simulink model "heading_controller"  (R2017b)
settings: Solver=ode45  StartTime=tstart  StopTime=tstop  RelTol=1e-3  EnableMultiTasking=on
values from neighbouring files (symbols this model uses):
  c = 0    [TTK4190_A3_task1_2.m]    (also in TTK4190_A3_task1_3.m = 1; model_analysis.m; msfartoystyring.m = sqrt(cun*ur*n + cnn*n^2); sysID.m)
  delta_max = 25*deg2rad    (= 0.436332312999)    [TTK4190_A3_task1_3.m]    (also in msfartoystyring.m)
  delta_min = -25*deg2rad    (= -0.436332312999)    [TTK4190_A3_task1_3.m]
  Kd_psi = 650    [TTK4190_A3_task1_3.m]    (also in parameters_heading_controller.m = 150)
  Ki_psi = 0.07    [TTK4190_A3_task1_3.m]    (also in parameters_heading_controller.m = 0.0004)
  Kp_psi = 60    [TTK4190_A3_task1_3.m]    (also in parameters_heading_controller.m = 0.8)
  nc = 7.3    [TTK4190_A3_task1_2.m]    (also in TTK4190_A3_task1_3.m; model_analysis.m; parameters_heading_controller.m; sysID.m)
  p0 = zeros(2,1)    [TTK4190_A3_task1_2.m]    (also in TTK4190_A3_task1_3.m; model_analysis.m; sysID.m)
  psi0 = 0    [TTK4190_A3_task1_2.m]    (also in TTK4190_A3_task1_3.m; model_analysis.m; sysID.m)
  psi_amp = -0.3    [TTK4190_A3_task1_3.m]
  psi_d = 5*deg2rad    (= 0.0872664625997)    [TTK4190_A3_task1_2.m]    (also in TTK4190_A3_task1_3.m = 0.13962634016; model_analysis.m = 0.13962634016; parameters_heading_controller.m = 0.13962634016)
  psi_freq = 0.008    [TTK4190_A3_task1_3.m]
  r0 = 0    [TTK4190_A3_task1_2.m]    (also in TTK4190_A3_task1_3.m; model_analysis.m; sysID.m)
  tsamp = 10    [TTK4190_A3_task1_2.m]    (also in TTK4190_A3_task1_3.m; model_analysis.m = 35; sim_nomoto2.m = tsamp; sysID.m = 100)
  v0 = [6.63 0]'    [TTK4190_A3_task1_2.m]    (also in TTK4190_A3_task1_3.m; model_analysis.m; sysID.m)
undefined symbols (not defined in the file or in its folder): msfartoystyring
settings Model: ExtModeAutoUpdateStatusClock=off  Creator=christh  LastModifiedBy=Marie
settings DataIOCC: LimitDataPoints=on  SaveFormat=Array  SignalLoggingSaveFormat=ModelDataLogs
settings OptimizationCC: ExpressionDepthLimit=2147483647  InitFltsAndDblsToZero=on  LifeSpan=inf
settings DebuggingCC: UnderspecifiedInitializationDetection=Classic  MergeDetectMultiDrivingBlocksExec=none  SolverPrmCheckMsg=warning  FcnCallInpInsideContextMsg=warning  StateNameClashWarn=warning  SFUnexpectedBacktrackingDiag=warning  SFNoUnconditionalDefaultTransitionDiag=warning  SFExecutionAtInitializationDiag=none
settings HardwareCC: ProdBitPerPointer=32  ProdBitPerSizeT=32  ProdBitPerPtrDiffT=32  ProdLargestAtomicFloat=None  ProdIntDivRoundTo=Undefined  ProdEndianess=Unspecified  ProdWordSize=32  ProdHWDeviceType=32-bit Generic
settings ModelReferenceCC: PropagateSignalLabelsOutOfModel=off
settings CodeAppCC: StateflowObjectComments=on
settings GRTTargetCC: TargetLangStandard=C89/C90 (ANSI)  GeneratePreprocessorConditionals=Disable all  CombineOutputUpdateFcns=off  GRTInterface=on
settings ConfigComp: CovMetricSettings=dw  CovHtmlReporting=on  CovSaveCumulativeToWorkspaceVar=on  CovSaveSingleToWorkspaceVar=on  CovExternalEMLEnable=off

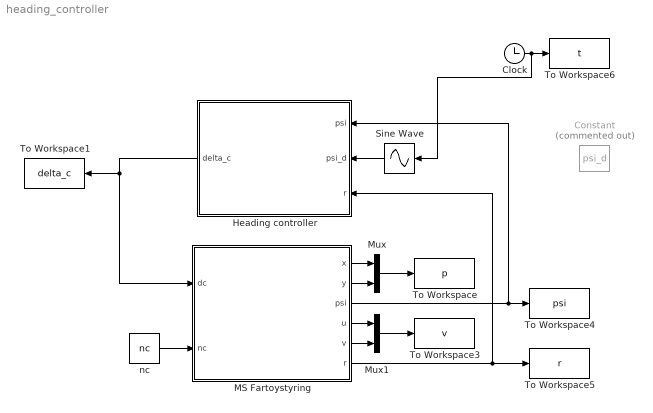
== system heading_controller ==
  Clock : Clock
  Constant : Constant  Commented=on  Value=psi_d
  Heading controller : Subsystem
  MS Fartoystyring : Subsystem  mask(MS Fartoystyring for Assignment 3 G&C){x0=p0(1), y0=p0(2), u0=v0(1), v0=v0(2), psi0=psi0, r0=r0, c=c}
      mask prompts: x0 "x(t0) (m)"; y0 "y(t0) (m)"; u0 "u(t0) (m/s)"; v0 "v(t0) (m/s)"; psi0 "psi(t0) (rad)"; r0 "r(t0) (rad/s)"; c "current (0 or 1)"
      mask help:
      | Block corresponding to Figure 1 in the assignment text. Gives the response of the ship.
      |
      | The design speed of MS Fartoystyring is u=8.23 m/s.
      |
      | Input:
      | dc: commanded rudder (rad), dmax=25*pi/180
      | nc: commanded shaft speed (rad/s), nmax=85*2*pi/60
      |
      | Output:
      | x: north pos (m)
      | y: east pos (m)
      | u: surge (m/s)
      | v: sway (m/s)
      | psi: heading (rad)
      | r: yaw (rad/s)
      mask Help: Comments, bugs and help requests can be directed to the TA. Email on course website.
  Mux : Mux  Inputs=2
  Mux1 : Mux  Inputs=2
  Sine Wave : Sin  TimeSource=Use external signal  Amplitude=psi_amp  Frequency=psi_freq  SampleTime=0
  To Workspace : ToWorkspace  VariableName=p  SampleTime=tsamp
  To Workspace1 : ToWorkspace  VariableName=delta_c  SampleTime=tsamp
  To Workspace3 : ToWorkspace  VariableName=v  SampleTime=tsamp
  To Workspace4 : ToWorkspace  VariableName=psi  SampleTime=tsamp
  To Workspace5 : ToWorkspace  VariableName=r  SampleTime=tsamp
  To Workspace6 : ToWorkspace  VariableName=t  SampleTime=tsamp
  nc : Constant  Value=nc
  wires:
  Clock/1 -> Sine Wave/1, To Workspace6/1
  MS Fartoystyring/1(x) -> Mux/1
  MS Fartoystyring/2(y) -> Mux/2
  MS Fartoystyring/4(u) -> Mux1/1
  MS Fartoystyring/5(v) -> Mux1/2
  Mux/1 -> To Workspace/1
  Mux1/1 -> To Workspace3/1
  MS Fartoystyring/3(psi) -> To Workspace4/1, Heading controller/1(psi)
  MS Fartoystyring/6(r) -> Heading controller/3(r), To Workspace5/1
  nc/1 -> MS Fartoystyring/2(nc)
  Heading controller/1(delta_c) -> MS Fartoystyring/1(dc), To Workspace1/1
  Sine Wave/1 -> Heading controller/2("psi_d ")

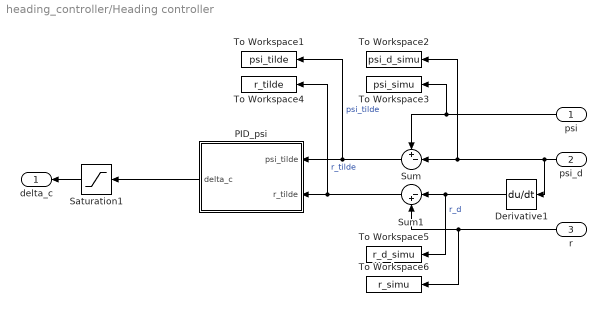
== system heading_controller/Heading controller ==
  psi : Inport
  "psi_d " : Inport  Port=2
  r : Inport  Port=3
  Derivative1 : Derivative
  PID_psi : Subsystem
  Saturation1 : Saturate  UpperLimit=delta_max  LowerLimit=delta_min
  Sum : Sum  Inputs=+-|
  Sum1 : Sum  Inputs=|-+
  To Workspace1 : ToWorkspace  VariableName=psi_tilde  SampleTime=tsamp
  To Workspace2 : ToWorkspace  VariableName=psi_d_simu  SampleTime=tsamp
  To Workspace3 : ToWorkspace  VariableName=psi_simu  SampleTime=tsamp
  To Workspace4 : ToWorkspace  VariableName=r_tilde  SampleTime=tsamp
  To Workspace5 : ToWorkspace  VariableName=r_d_simu  SampleTime=tsamp
  To Workspace6 : ToWorkspace  VariableName=r_simu  SampleTime=tsamp
  delta_c : Outport
  wires:
  "psi_d "/1 -> To Workspace2/1, Sum/2, Derivative1/1
  Sum1/1 -> To Workspace4/1, PID_psi/2(r_tilde)  "r_tilde"
  Derivative1/1 -> To Workspace5/1, Sum1/1  "r_d"
  Sum/1 -> To Workspace1/1, PID_psi/1(psi_tilde)  "psi_tilde"
  r/1 -> To Workspace6/1, Sum1/2
  PID_psi/1(delta_c) -> Saturation1/1
  Saturation1/1 -> delta_c/1
  psi/1 -> To Workspace3/1, Sum/1

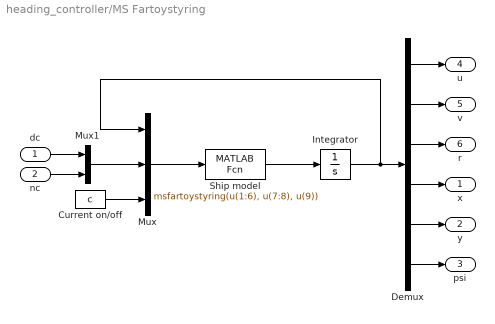
== system heading_controller/MS Fartoystyring ==
  dc : Inport
  nc : Inport  Port=2
  Current on/off : Constant  Value=c
  Demux : Demux  Outputs=6
  Integrator : Integrator  InitialCondition=[u0 v0 r0 x0 y0 psi0]'
  Mux : Mux  Inputs=3
  Mux1 : Mux  Inputs=2
  Ship model : MATLABFcn  MATLABFcn=msfartoystyring(u(1:6), u(7:8), u(9))  OutputDimensions=6
  x : Outport
  y : Outport  Port=2
  psi : Outport  Port=3
  u : Outport  Port=4
  v : Outport  Port=5
  r : Outport  Port=6
  wires:
  Integrator/1 -> Mux/1, Demux/1
  Mux1/1 -> Mux/2
  dc/1 -> Mux1/1
  nc/1 -> Mux1/2
  Demux/1 -> u/1
  Demux/2 -> v/1
  Demux/3 -> r/1
  Demux/4 -> x/1
  Demux/5 -> y/1
  Demux/6 -> psi/1
  Current on/off/1 -> Mux/3
  Ship model/1 -> Integrator/1
  Mux/1 -> Ship model/1

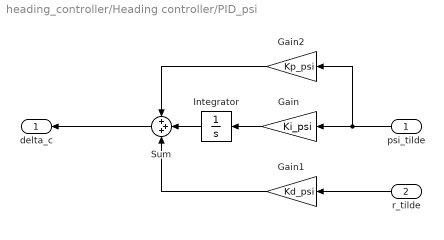
== system heading_controller/Heading controller/PID_psi ==
  psi_tilde : Inport
  r_tilde : Inport  Port=2
  Gain : Gain  Gain=Ki_psi
  Gain1 : Gain  Gain=Kd_psi
  Gain2 : Gain  Gain=Kp_psi
  Integrator : Integrator
  Sum : Sum  Inputs=+++
  delta_c : Outport
  wires:
  Gain2/1 -> Sum/1
  r_tilde/1 -> Gain1/1
  Gain1/1 -> Sum/3
  psi_tilde/1 -> Gain2/1, Gain/1
  Sum/1 -> delta_c/1
  Gain/1 -> Integrator/1
  Integrator/1 -> Sum/2
